simulink model "lab7"  (R2019a)
settings: Solver=VariableStepAuto  StartTime=0.0  StopTime=500  RelTol=1e-3
settings Model: Creator=sumli  LastModifiedBy=sumli

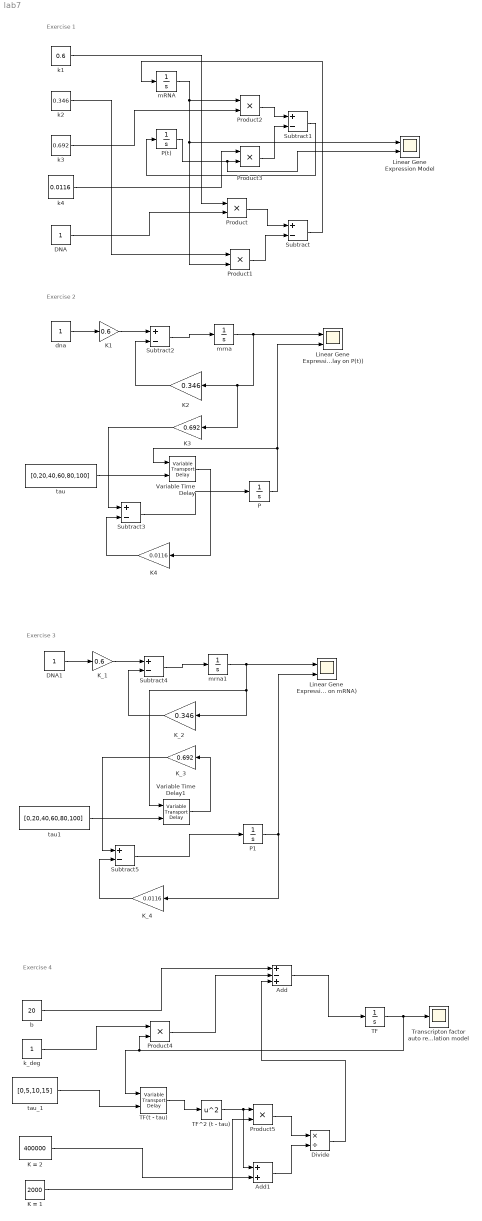
== system lab7 ==
  note: Exercise 4
  note: Exercise 3
  note: Exercise 2
  note: Exercise 1
  Add : Sum  Inputs=+-+
  Add1 : Sum
  DNA : Constant
  DNA1 : Constant
  Divide : Product  Inputs=*/
  K = 1 : Constant  Value=2000
  K = 2 : Constant  Value=400000
  K1 : Gain  Gain=0.6
  K2 : Gain  Gain=0.346
  K3 : Gain  Gain=0.692
  K4 : Gain  Gain=0.0116
  K_1 : Gain  Gain=0.6
  K_2 : Gain  Gain=0.346
  K_3 : Gain  Gain=0.692
  K_4 : Gain  Gain=0.0116
  Linear Gene Expression Model : Scope  NumInputPorts=2
  Linear Gene Expression Model (Time Delay on P(t)) : Scope  NumInputPorts=2
  Linear Gene Expression Model (Time Delay on mRNA) : Scope  NumInputPorts=2
  P : Integrator
  P(t) : Integrator
  P1 : Integrator
  Product{,1..5} (6 alike) : Product
  Subtract{,1..5} (6 alike) : Sum  Inputs=+-
  TF : Integrator  InitialCondition=200
  TF(t - tau) : VariableTransportDelay  MaximumDelay=15  InitialOutput=200
  TF^2 (t - tau) : Math  Operator=square  SaturateOnIntegerOverflow=on
  Transcripton factor auto regulation model : Scope
  Variable Time Delay : VariableTransportDelay  MaximumDelay=200
  Variable Time Delay1 : VariableTransportDelay  MaximumDelay=200
  b : Constant  Value=20
  dna : Constant
  k1 : Constant  Value=0.6
  k2 : Constant  Value=0.346
  k3 : Constant  Value=0.692
  k4 : Constant  Value=0.0116
  k_deg : Constant
  mRNA : Integrator
  mrna : Integrator
  mrna1 : Integrator
  tau : Constant  Value=[0,20,40,60,80,100]
  tau1 : Constant  Value=[0,20,40,60,80,100]
  tau_1 : Constant  Value=[0,5,10,15]
  wires:
  DNA/1 -> Product/2
  k1/1 -> Product/1
  k2/1 -> Product1/1
  mRNA/1 -> Product1/2, Linear Gene Expression Model/1, Product2/1
  Product/1 -> Subtract/1
  Product1/1 -> Subtract/2
  k3/1 -> Product2/2
  k4/1 -> Product3/1
  P(t)/1 -> Linear Gene Expression Model/2, Product3/2
  Product2/1 -> Subtract1/1
  Product3/1 -> Subtract1/2
  Subtract/1 -> mRNA/1
  Subtract1/1 -> P(t)/1
  Subtract2/1 -> mrna/1
  mrna/1 -> K3/1, K2/1, Linear Gene Expression Model (Time Delay on P(t))/1
  K2/1 -> Subtract2/2
  dna/1 -> K1/1
  K1/1 -> Subtract2/1
  P/1 -> Variable Time Delay/1, Linear Gene Expression Model (Time Delay on P(t))/2
  Subtract3/1 -> P/1
  Variable Time Delay/1 -> K4/1
  K4/1 -> Subtract3/2
  K3/1 -> Subtract3/1
  tau/1 -> Variable Time Delay/2
  DNA1/1 -> K_1/1
  K_1/1 -> Subtract4/1
  tau1/1 -> Variable Time Delay1/2
  K_2/1 -> Subtract4/2
  mrna1/1 -> Variable Time Delay1/1, K_2/1, Linear Gene Expression Model (Time Delay on mRNA)/1
  Subtract4/1 -> mrna1/1
  K_3/1 -> Subtract5/1
  K_4/1 -> Subtract5/2
  Variable Time Delay1/1 -> K_3/1
  Subtract5/1 -> P1/1
  P1/1 -> Linear Gene Expression Model (Time Delay on mRNA)/2, K_4/1
  tau_1/1 -> TF(t - tau)/2
  TF/1 -> TF(t - tau)/1, Product4/2, Transcripton factor auto regulation model/1
  Add/1 -> TF/1
  k_deg/1 -> Product4/1
  b/1 -> Add/1
  TF(t - tau)/1 -> TF^2 (t - tau)/1
  TF^2 (t - tau)/1 -> Add1/1, Product5/1
  Product5/1 -> Divide/1
  Add1/1 -> Divide/2
  Divide/1 -> Add/3
  Product4/1 -> Add/2
  K = 1/1 -> Product5/2
  K = 2/1 -> Add1/2
